simulink model "Torque_Vectoring_2_Wheelspeed"  (R2015b)
settings: Solver=VariableStepAuto  StartTime=0.0  StopTime=10.0  RelTol=1e-3
undefined symbols (not defined in the file or in its folder): magnitude
settings Model: Creator=Niels  LastModifiedBy=Niels

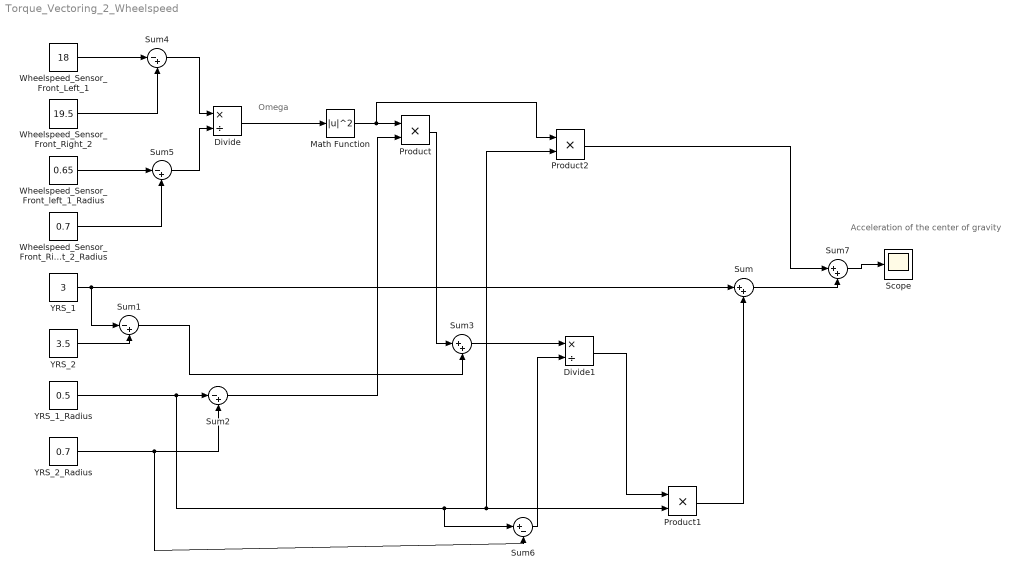
== system Torque_Vectoring_2_Wheelspeed ==
  note: Acceleration of the center of gravity
  note: Omega
  Divide : Product  Inputs=*/
  Divide1 : Product  Inputs=*/
  Math Function : Math  Operator=magnitude^2  SaturateOnIntegerOverflow=on
  Product : Product
  Product1 : Product
  Product2 : Product
  Scope : Scope
  Sum : Sum  Inputs=|++
  Sum{1..2,4..5} (4 alike) : Sum  Inputs=|-+
  Sum3 : Sum  Inputs=|++
  Sum6 : Sum  Inputs=|+-
  Sum7 : Sum  Inputs=|++
  Wheelspeed_Sensor_Front_Left_1 : Constant  Value=18
  Wheelspeed_Sensor_Front_Right_2 : Constant  Value=19.5
  Wheelspeed_Sensor_Front_Right_2_Radius : Constant  Value=0.7
  Wheelspeed_Sensor_Front_left_1_Radius : Constant  Value=0.65
  "YRS_1 " : Constant  Value=3
  YRS_1_Radius : Constant  Value=0.5
  YRS_2 : Constant  Value=3.5
  YRS_2_Radius : Constant  Value=0.7
  wires:
  "YRS_1 "/1 -> Sum1/1, Sum/1
  YRS_1_Radius/1 -> Product2/2, Product1/2, Sum6/1, Sum2/1
  YRS_2/1 -> Sum1/2
  YRS_2_Radius/1 -> Sum6/2, Sum2/2
  Wheelspeed_Sensor_Front_Left_1/1 -> Sum4/1
  Wheelspeed_Sensor_Front_Right_2/1 -> Sum4/2
  Wheelspeed_Sensor_Front_Right_2_Radius/1 -> Sum5/2
  Wheelspeed_Sensor_Front_left_1_Radius/1 -> Sum5/1
  Sum4/1 -> Divide/1
  Sum5/1 -> Divide/2
  Divide/1 -> Math Function/1
  Math Function/1 -> Product2/1, Product/1
  Sum2/1 -> Product/2
  Product/1 -> Sum3/1
  Sum1/1 -> Sum3/2
  Sum3/1 -> Divide1/1
  Sum6/1 -> Divide1/2
  Divide1/1 -> Product1/1
  Product1/1 -> Sum/2
  Product2/1 -> Sum7/1
  Sum/1 -> Sum7/2
  Sum7/1 -> Scope/1
